simulink model "pendulo_invertido"  (R2023a)
settings: Solver=ode45  StartTime=0.0  StopTime=10  RelTol=1e-3
values from neighbouring files (symbols this model uses):
  Beq = 4.3    [practica_1_sdmyss.m]
  Bp = 0.0024    [practica_1_sdmyss.m]
  Fc = 0    [practica_1_sdmyss.m]
  g = 9.81    [practica_1_sdmyss.m]
  Ip = 0.0079    [practica_1_sdmyss.m]
  lp = 0.3302    [practica_1_sdmyss.m]
  Mc = 0.7031    [practica_1_sdmyss.m]
  Mp = 0.23    [practica_1_sdmyss.m]
undefined symbols (not defined in the file or in its folder): magnitude
settings Model: Creator=danie  LastModifiedBy=danie

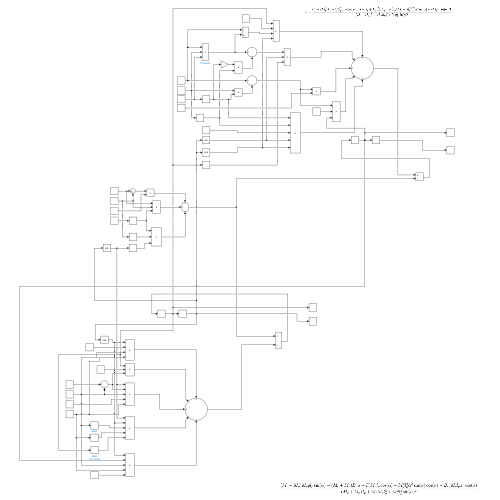
[thumbnail: Simulink's stored preview of the top-level diagram]
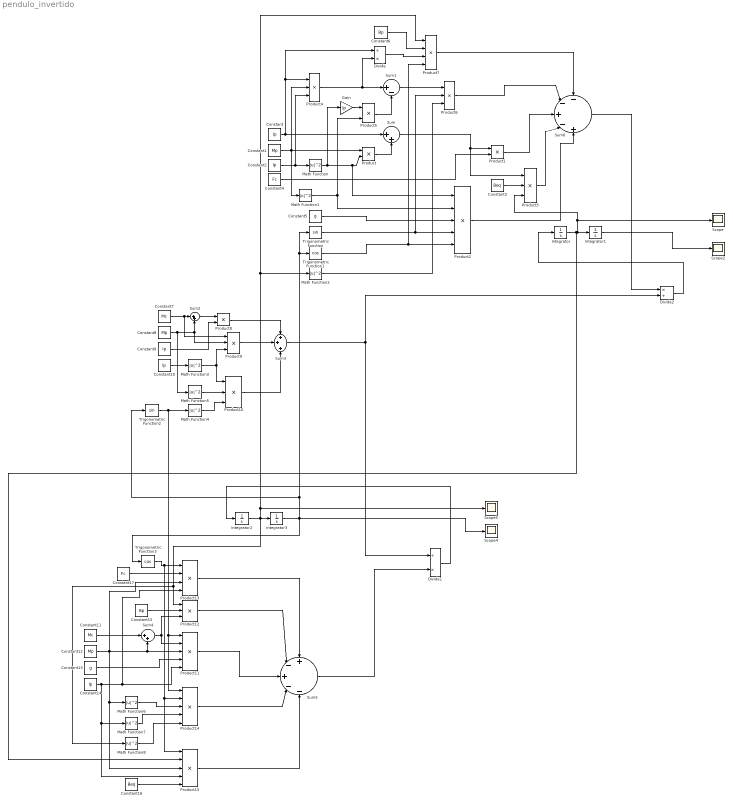
== system pendulo_invertido ==
  Constant : Constant  Value=Ip
  Constant1 : Constant  Value=Mp
  Constant10 : Constant  Value=lp
  Constant11 : Constant  Value=Mc
  Constant12 : Constant  Value=Mp
  Constant13 : Constant  Value=g
  Constant14 : Constant  Value=lp
  Constant15 : Constant  Value=Bp
  Constant16 : Constant  Value=Beq
  Constant17 : Constant  Value=Fc
  Constant2 : Constant  Value=lp
  Constant3 : Constant  Value=Beq
  Constant4 : Constant  Value=Fc
  Constant5 : Constant  Value=g
  Constant6 : Constant  Value=Bp
  Constant7 : Constant  Value=Mc
  Constant8 : Constant  Value=Mp
  Constant9 : Constant  Value=Ip
  Divide : Product  Inputs=/*
  Divide1 : Product  Inputs=/*
  Divide2 : Product  Inputs=*/
  Gain : Gain  Gain=lp
  Integrator : Integrator
  Integrator1 : Integrator
  Integrator2 : Integrator
  Integrator3 : Integrator  InitialCondition=1*pi/180
  Math Function{,1..8} (9 alike) : Math  Operator=magnitude^2
  Product{,1,5,8} (4 alike) : Product
  Product{3..4,6,9..10,12} (6 alike) : Product  Inputs=3
  Product{2,11,14..15} (4 alike) : Product  Inputs=5
  Product13 : Product  Inputs=4
  Product7 : Product  Inputs=4
  Scope{,2,4..5} (4 alike) : Scope
  Sum : Sum  Inputs=|++
  Sum1 : Sum  Inputs=|+-
  Sum2 : Sum  Inputs=|++
  Sum3 : Sum  Inputs=+++
  Sum4 : Sum  Inputs=|++
  Sum5 : Sum  Inputs=+-+--
  Sum6 : Sum  Inputs=--+-+
  Trigonometric Function : Trigonometry
  Trigonometric Function1 : Trigonometry  Operator=cos
  Trigonometric Function2 : Trigonometry
  Trigonometric Function3 : Trigonometry  Operator=cos
  wires:
  Integrator/1 -> Product15/2, Scope/1, Product3/3, Integrator1/1
  Integrator2/1 -> Math Function8/1, Product12/1, Scope5/1, Math Function2/1, Product7/1, Integrator3/1
  Constant1/1 -> Product/1, Math Function1/1, Product4/2
  Constant2/1 -> Product4/3, Math Function/1
  Math Function/1 -> Gain/1, Product2/1, Product/2
  Constant/1 -> Divide/1, Product4/1, Sum/1
  Product/1 -> Sum/2
  Sum/1 -> Product3/1, Product1/1
  Constant4/1 -> Product1/2
  Math Function1/1 -> Product5/2, Product2/2
  Constant5/1 -> Product2/3
  Trigonometric Function/1 -> Product6/2, Product2/4
  Trigonometric Function1/1 -> Product7/4, Product2/5
  Integrator3/1 -> Trigonometric Function3/1, Scope4/1, Trigonometric Function/1, Trigonometric Function1/1, Trigonometric Function2/1
  Constant3/1 -> Product3/2
  Gain/1 -> Product5/1
  Product5/1 -> Sum1/2
  Product4/1 -> Divide/2, Sum1/1
  Math Function2/1 -> Product6/3
  Sum1/1 -> Product6/1
  Divide/1 -> Product7/3
  Constant6/1 -> Product7/2
  Constant7/1 -> Product9/1, Sum2/1
  Constant8/1 -> Math Function5/1, Product9/2, Sum2/2
  Sum2/1 -> Product8/1
  Constant9/1 -> Product8/2
  Constant10/1 -> Math Function3/1
  Math Function3/1 -> Product10/1, Product9/3
  Trigonometric Function2/1 -> Math Function4/1, Product11/1, Product14/1
  Math Function5/1 -> Product10/2
  Math Function4/1 -> Product10/3
  Product9/1 -> Sum3/2
  Product8/1 -> Sum3/1
  Product10/1 -> Sum3/3
  Constant11/1 -> Sum4/1
  Constant12/1 -> Product15/3, Math Function6/1, Sum4/2, Product11/3, Product13/3
  Constant14/1 -> Product13/4, Product11/5, Product15/4, Math Function7/1
  Constant13/1 -> Product11/4
  Sum4/1 -> Product12/3, Product11/2
  Constant15/1 -> Product12/2
  Trigonometric Function3/1 -> Product14/2, Product15/1, Product13/1
  Constant17/1 -> Product13/2
  Math Function8/1 -> Product14/5
  Math Function7/1 -> Product14/4
  Math Function6/1 -> Product14/3
  Constant16/1 -> Product15/5
  Product15/1 -> Sum5/5
  Product14/1 -> Sum5/4
  Product11/1 -> Sum5/3
  Product12/1 -> Sum5/2
  Product13/1 -> Sum5/1
  Sum5/1 -> Divide1/2
  Sum3/1 -> Divide2/2, Divide1/1
  Divide1/1 -> Integrator2/1
  Product7/1 -> Sum6/1
  Product6/1 -> Sum6/2
  Product1/1 -> Sum6/3
  Product2/1 -> Sum6/5
  Product3/1 -> Sum6/4
  Sum6/1 -> Divide2/1
  Divide2/1 -> Integrator/1
  Integrator1/1 -> Scope2/1
